simulink model "motor"  (Simulink 7.1)
settings: Solver=ode1  StartTime=0.0  StopTime=10.0  FixedStep=h  RelTol=1e-3
undefined symbols (not defined in the file or in its folder): B, J, ka, kc, kg, kt, La, Ra
settings Model: Creator=jacoud  LastModifiedBy=jacoud
settings DataIOCC: SignalLoggingName=sigsOut
settings DebuggingCC: SaveWithParameterizedLinksMsg=none  SignalResolutionControl=TryResolveAllWithWarning  SolverPrmCheckMsg=none  MultiTaskDSMMsg=warning  MultiTaskCondExecSysMsg=none  StrictBusMsg=None
settings HardwareCC: TargetUnknown=on
settings RTWCC: IncludeERTFirstTime=on

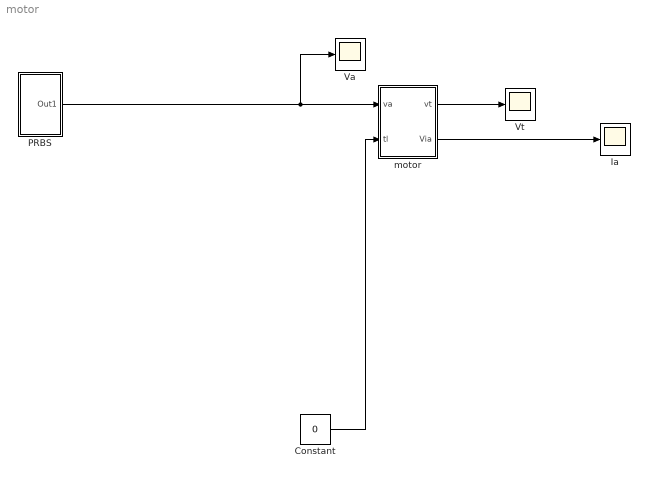
== system motor ==
  Constant : Constant  Value=0  OutDataType=sfix(16)  OutScaling=2^0
  Ia : Scope
      settings: SaveName=dadosia
  PRBS : Subsystem
  Va : Scope
      settings: SaveName=dadosva
  Vt : Scope
      settings: SaveName=dadosvt
  motor : Subsystem
  wires:
  Constant/1 -> motor/2(tl)
  motor/2(Via) -> Ia/1
  motor/1(vt) -> Vt/1
  PRBS/1(Out1) -> motor/1(va), Va/1

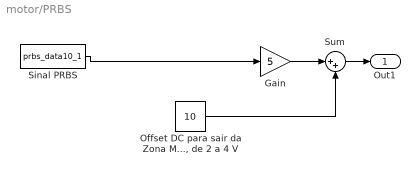
== system motor/PRBS ==
  Gain : Gain  Gain=5  ParameterDataType=sfix(16)  ParameterScaling=2^0  OutDataType=sfix(16)  OutScaling=2^0  SaturateOnIntegerOverflow=on  OutDataTypeStr=Inherit: Same as input  ParamDataTypeStr=Inherit: Same as input
  "Offset DC para sair da Zona Morta Variando, agora, de 2 a 4 V " : Constant  Value=10  OutDataType=sfix(16)  OutScaling=2^0
  Sinal PRBS : FromWorkspace  VariableName=prbs_data10_1  SampleTime=0  OutputAfterFinalValue=Holding final value
  Sum : Sum  Inputs=|++  OutDataType=sfix(16)  OutScaling=2^0  SaturateOnIntegerOverflow=on
  Out1 : Outport
  wires:
  Sinal PRBS/1 -> Gain/1
  "Offset DC para sair da Zona Morta Variando, agora, de 2 a 4 V "/1 -> Sum/2
  Gain/1 -> Sum/1
  Sum/1 -> Out1/1

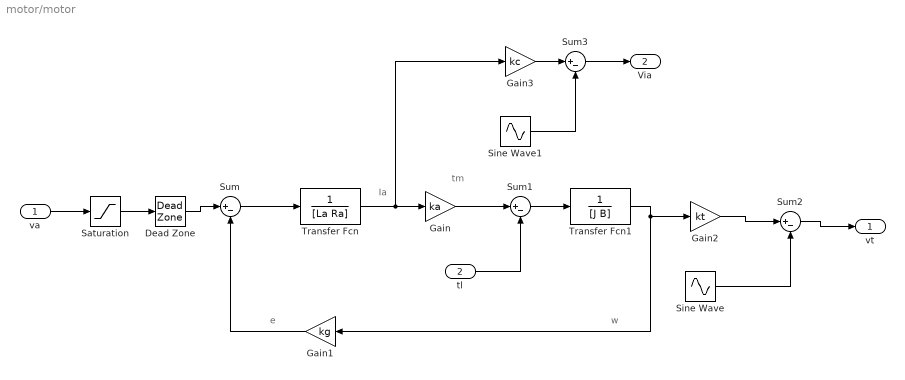
== system motor/motor ==
  note: Ia
  note: tm
  note: e
  note: w
  va : Inport  OutDataType=sfix(16)  OutScaling=2^0
  tl : Inport  Port=2  OutDataType=sfix(16)  OutScaling=2^0
  Dead Zone : DeadZone  LowerValue=-1  UpperValue=1  SaturateOnIntegerOverflow=on
  Gain : Gain  Gain=ka  ParameterDataType=sfix(16)  ParameterScaling=2^0  OutDataType=sfix(16)  OutScaling=2^0  SaturateOnIntegerOverflow=on  OutDataTypeStr=Inherit: Same as input  ParamDataTypeStr=Inherit: Same as input
  Gain1 : Gain  Orientation=left  Gain=kg  ParameterDataType=sfix(16)  ParameterScaling=2^0  OutDataType=sfix(16)  OutScaling=2^0  SaturateOnIntegerOverflow=on  OutDataTypeStr=Inherit: Same as input  ParamDataTypeStr=Inherit: Same as input
  Gain2 : Gain  Gain=kt  ParameterDataType=sfix(16)  ParameterScaling=2^0  OutDataType=sfix(16)  OutScaling=2^0  SaturateOnIntegerOverflow=on  OutDataTypeStr=Inherit: Same as input  ParamDataTypeStr=Inherit: Same as input
  Gain3 : Gain  Gain=kc  ParameterDataType=sfix(16)  ParameterScaling=2^0  OutDataType=sfix(16)  OutScaling=2^0  SaturateOnIntegerOverflow=on  OutDataTypeStr=Inherit: Same as input  ParamDataTypeStr=Inherit: Same as input
  Saturation : Saturate  UpperLimit=20  LowerLimit=-20
  Sine Wave : Sin  Amplitude=0.2  Frequency=2*pi*50  SampleTime=0
  Sine Wave1 : Sin  Amplitude=0.1  Frequency=2*pi*50  SampleTime=0
  Sum{,1..3} (4 alike) : Sum  Inputs=|+-  OutDataType=sfix(16)  OutScaling=2^0  SaturateOnIntegerOverflow=on
  Transfer Fcn : TransferFcn  Denominator=[La Ra]
  Transfer Fcn1 : TransferFcn  Denominator=[J B]
  vt : Outport
  Via : Outport  Port=2
  wires:
  Sum/1 -> Transfer Fcn/1
  Transfer Fcn/1 -> Gain/1, Gain3/1
  Gain/1 -> Sum1/1
  Sum1/1 -> Transfer Fcn1/1
  Transfer Fcn1/1 -> Gain1/1, Gain2/1
  Gain1/1 -> Sum/2
  tl/1 -> Sum1/2
  Sine Wave/1 -> Sum2/2
  Gain3/1 -> Sum3/1
  Sine Wave1/1 -> Sum3/2
  Sum3/1 -> Via/1
  va/1 -> Saturation/1
  Dead Zone/1 -> Sum/1
  Saturation/1 -> Dead Zone/1
  Gain2/1 -> Sum2/1
  Sum2/1 -> vt/1
